simulink model "Indexer"  (R2018b)
settings: Solver=ode1  StartTime=0.0  StopTime=10.0  FixedStep=0.001  RelTol=1e-3
undefined symbols (not defined in the file): world
libraries: simulink x7
settings Model: Creator=ogihara  LastModifiedBy=ogihara

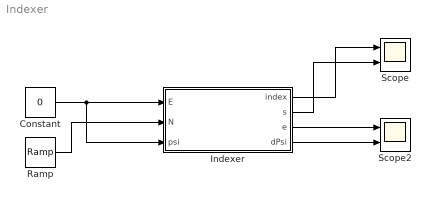
== system Indexer ==
  Constant : Constant  Value=0
  Indexer : Subsystem
  Ramp : simulink/Sources/Ramp  slope=10  start=0  InitialOutput=0
  Scope : Scope  NumInputPorts=2
  Scope2 : Scope  NumInputPorts=2
  wires:
  Constant/1 -> Indexer/3(psi), Indexer/1(E)
  Ramp/1 -> Indexer/2(N)
  Indexer/3(e) -> Scope2/1
  Indexer/4(dPsi) -> Scope2/2
  Indexer/1(index) -> Scope/1
  Indexer/2(s) -> Scope/2

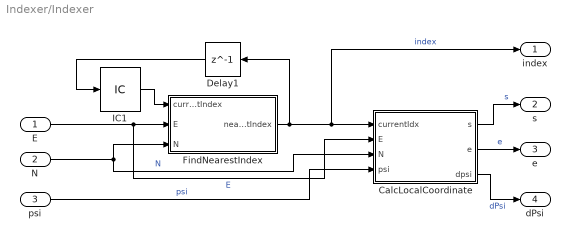
== system Indexer/Indexer ==
  E : Inport
  N : Inport  Port=2
  psi : Inport  Port=3
  CalcLocalCoordinate : Subsystem
  Delay1 : Delay  DelayLength=1
  FindNearestIndex : Subsystem
  IC1 : InitialCondition
  index : Outport
  s : Outport  Port=2
  e : Outport  Port=3
  dPsi : Outport  Port=4
  wires:
  IC1/1 -> FindNearestIndex/1(currentIndex)
  CalcLocalCoordinate/3(dpsi) -> dPsi/1  "dPsi"
  FindNearestIndex/1(nearestIndex) -> index/1, CalcLocalCoordinate/1(currentIdx), Delay1/1  "index"
  psi/1 -> CalcLocalCoordinate/4(psi)  "psi"
  E/1 -> CalcLocalCoordinate/2(E), FindNearestIndex/2(E)  "E"
  Delay1/1 -> IC1/1
  CalcLocalCoordinate/1(s) -> s/1  "s"
  N/1 -> CalcLocalCoordinate/3(N), FindNearestIndex/3(N)  "N"
  CalcLocalCoordinate/2(e) -> e/1  "e"

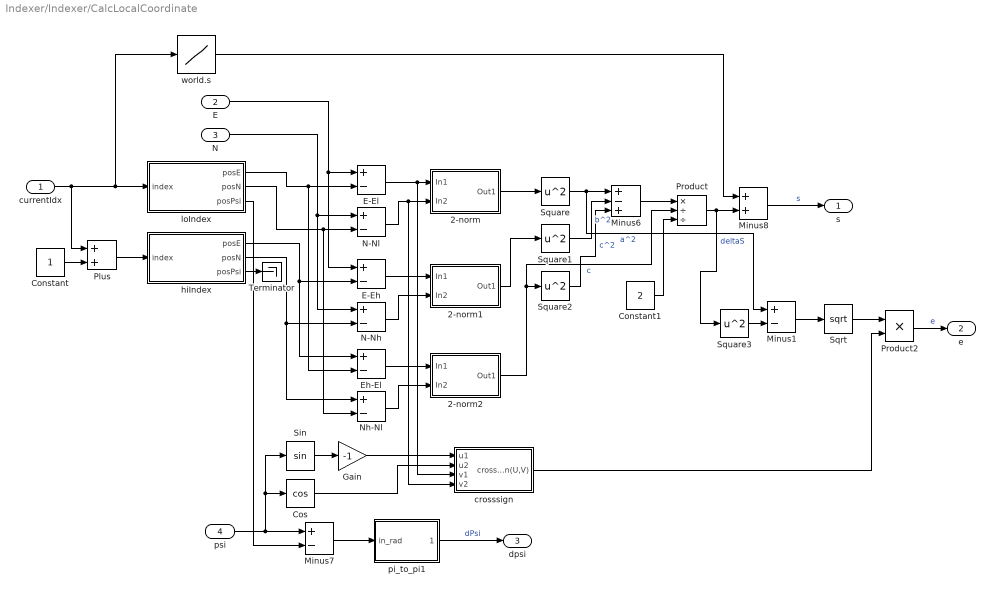
== system Indexer/Indexer/CalcLocalCoordinate ==
  currentIdx : Inport
  E : Inport  Port=2
  N : Inport  Port=3
  psi : Inport  Port=4
  2-norm : Subsystem
  2-norm1 : Subsystem
  2-norm2 : Subsystem
  Constant : Constant
  Constant1 : Constant  Value=2
  Cos : Trigonometry  Operator=cos
  E-Eh : Sum  Inputs=+-
  E-El : Sum  Inputs=+-
  Eh-El : Sum  Inputs=+-
  Gain : Gain  Gain=-1
  Minus1 : Sum  Inputs=+-
  Minus6 : Sum  Inputs=+-+
  Minus7 : Sum  Inputs=+-
  Minus8 : Sum
  N-Nh : Sum  Inputs=+-
  N-Nl : Sum  Inputs=+-
  Nh-Nl : Sum  Inputs=+-
  Plus : Sum
  Product : Product  Inputs=*//
  Product2 : Product
  Sin : Trigonometry
  Sqrt : Sqrt  SaturateOnIntegerOverflow=on
  Square{,1..3} (4 alike) : Math  Operator=square  SaturateOnIntegerOverflow=on
  Terminator : Terminator
  crosssign : Subsystem
  hiIndex : Subsystem
  loIndex : Subsystem
  pi_to_pi1 : Subsystem
  world.s : Lookup_n-D  NumberOfTableDimensions=1  BreakpointsForDimension1=world.index  Table=world.s_m  InternalRulePriority=Speed  RndMeth=Simplest  InputSameDT=on
  s : Outport
  e : Outport  Port=2
  dpsi : Outport  Port=3
  wires:
  currentIdx/1 -> Plus/1, world.s/1, loIndex/1(index)
  Constant/1 -> Plus/2
  Plus/1 -> hiIndex/1(index)
  hiIndex/3(posPsi) -> Terminator/1
  hiIndex/1(posE) -> Eh-El/1, E-Eh/2
  E-El/1 -> crosssign/3(v1), 2-norm/1(In1)
  N-Nl/1 -> crosssign/4(v2), 2-norm/2(In2)
  E-Eh/1 -> 2-norm1/1(In1)
  N-Nh/1 -> 2-norm1/2(In2)
  Eh-El/1 -> 2-norm2/1(In1)
  Nh-Nl/1 -> 2-norm2/2(In2)
  2-norm/1(Out1) -> Square/1
  2-norm1/1(Out1) -> Square1/1
  2-norm2/1(Out1) -> Product/2, Square2/1  "c"
  Square/1 -> Minus1/1, Minus6/1  "a^2"
  Square1/1 -> Minus6/2  "b^2"
  Square2/1 -> Minus6/3  "c^2"
  Minus6/1 -> Product/1
  Constant1/1 -> Product/3
  psi/1 -> Cos/1, Sin/1, Minus7/1
  Minus7/1 -> pi_to_pi1/1(in_rad)
  Product/1 -> Square3/1, Minus8/2  "deltaS"
  world.s/1 -> Minus8/1
  Minus8/1 -> s/1  "s"
  Sin/1 -> Gain/1
  Gain/1 -> crosssign/1(u1)
  Cos/1 -> crosssign/2(u2)
  E/1 -> E-Eh/1, E-El/1
  loIndex/1(posE) -> Eh-El/2, E-El/2
  loIndex/2(posN) -> Nh-Nl/2, N-Nl/2
  N/1 -> N-Nh/1, N-Nl/1
  hiIndex/2(posN) -> Nh-Nl/1, N-Nh/2
  loIndex/3(posPsi) -> Minus7/2
  Square3/1 -> Minus1/2
  Minus1/1 -> Sqrt/1
  Sqrt/1 -> Product2/1
  Product2/1 -> e/1  "e"
  crosssign/1(crosssign(U,V)) -> Product2/2
  pi_to_pi1/1(out_rad) -> dpsi/1  "dPsi"

== system Indexer/Indexer/FindNearestIndex ==
  note: Osprey had forward & backward search.
      | This simulator has only forward search and max width is 5.
  currentIndex : Inport
  E : Inport  Port=2
  N : Inport  Port=3
  ForwardSearch : Subsystem  TreatAsAtomicUnit=on
  nearestIndex : Outport
  wires:
  currentIndex/1 -> ForwardSearch/1(CurrentIndex)
  E/1 -> ForwardSearch/2(E)
  N/1 -> ForwardSearch/3(N)
  ForwardSearch/1(loIndexF) -> nearestIndex/1

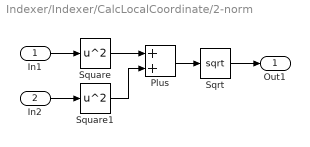
== system Indexer/Indexer/CalcLocalCoordinate/2-norm ==
  In1 : Inport
  In2 : Inport  Port=2
  Plus : Sum
  Sqrt : Sqrt  SaturateOnIntegerOverflow=on
  Square : Math  Operator=square  SaturateOnIntegerOverflow=on
  Square1 : Math  Operator=square  SaturateOnIntegerOverflow=on
  Out1 : Outport
  wires:
  In1/1 -> Square/1
  In2/1 -> Square1/1
  Square/1 -> Plus/1
  Square1/1 -> Plus/2
  Plus/1 -> Sqrt/1
  Sqrt/1 -> Out1/1

== system Indexer/Indexer/CalcLocalCoordinate/2-norm1 ==
  In1 : Inport
  In2 : Inport  Port=2
  Plus : Sum
  Sqrt : Sqrt  SaturateOnIntegerOverflow=on
  Square : Math  Operator=square  SaturateOnIntegerOverflow=on
  Square1 : Math  Operator=square  SaturateOnIntegerOverflow=on
  Out1 : Outport
  wires:
  In1/1 -> Square/1
  In2/1 -> Square1/1
  Square/1 -> Plus/1
  Square1/1 -> Plus/2
  Plus/1 -> Sqrt/1
  Sqrt/1 -> Out1/1

== system Indexer/Indexer/CalcLocalCoordinate/2-norm2 ==
  In1 : Inport
  In2 : Inport  Port=2
  Plus : Sum
  Sqrt : Sqrt  SaturateOnIntegerOverflow=on
  Square : Math  Operator=square  SaturateOnIntegerOverflow=on
  Square1 : Math  Operator=square  SaturateOnIntegerOverflow=on
  Out1 : Outport
  wires:
  In1/1 -> Square/1
  In2/1 -> Square1/1
  Square/1 -> Plus/1
  Square1/1 -> Plus/2
  Plus/1 -> Sqrt/1
  Sqrt/1 -> Out1/1

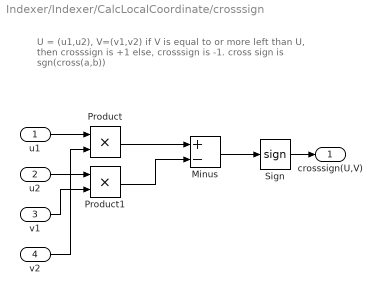
== system Indexer/Indexer/CalcLocalCoordinate/crosssign ==
  note: U = (u1,u2), V=(v1,v2)
      | if V is equal to or more left than U, then crosssign is +1
      | else, crosssign is -1.
      |
      | cross sign is sgn(cross(a,b))
  u1 : Inport
  u2 : Inport  Port=2
  v1 : Inport  Port=3
  v2 : Inport  Port=4
  Minus : Sum  Inputs=+-
  Product : Product
  Product1 : Product
  Sign : Signum
  crosssign(U,V) : Outport
  wires:
  Minus/1 -> Sign/1
  Sign/1 -> crosssign(U,V)/1
  u1/1 -> Product/1
  v2/1 -> Product/2
  u2/1 -> Product1/1
  v1/1 -> Product1/2
  Product/1 -> Minus/1
  Product1/1 -> Minus/2

== system Indexer/Indexer/CalcLocalCoordinate/hiIndex ==
  index : Inport
  world.posE_m : Lookup_n-D  NumberOfTableDimensions=1  BreakpointsForDimension1=world.index  Table=world.posE_m  InternalRulePriority=Speed  RndMeth=Simplest  InputSameDT=on
  world.posN_m : Lookup_n-D  NumberOfTableDimensions=1  BreakpointsForDimension1=world.index  Table=world.posN_m  InternalRulePriority=Speed  RndMeth=Simplest  InputSameDT=on
  world.psi_rad : Lookup_n-D  NumberOfTableDimensions=1  BreakpointsForDimension1=world.index  Table=world.psi_rad  InternalRulePriority=Speed  RndMeth=Simplest  InputSameDT=on
  posE : Outport
  posN : Outport  Port=2
  posPsi : Outport  Port=3
  wires:
  world.psi_rad/1 -> posPsi/1
  index/1 -> world.psi_rad/1, world.posN_m/1, world.posE_m/1
  world.posE_m/1 -> posE/1
  world.posN_m/1 -> posN/1

== system Indexer/Indexer/CalcLocalCoordinate/loIndex ==
  index : Inport
  world.posE_m : Lookup_n-D  NumberOfTableDimensions=1  BreakpointsForDimension1=world.index  Table=world.posE_m  InternalRulePriority=Speed  RndMeth=Simplest  InputSameDT=on
  world.posN_m : Lookup_n-D  NumberOfTableDimensions=1  BreakpointsForDimension1=world.index  Table=world.posN_m  InternalRulePriority=Speed  RndMeth=Simplest  InputSameDT=on
  world.psi_rad : Lookup_n-D  NumberOfTableDimensions=1  BreakpointsForDimension1=world.index  Table=world.psi_rad  InternalRulePriority=Speed  RndMeth=Simplest  InputSameDT=on
  posE : Outport
  posN : Outport  Port=2
  posPsi : Outport  Port=3
  wires:
  world.psi_rad/1 -> posPsi/1
  index/1 -> world.psi_rad/1, world.posN_m/1, world.posE_m/1
  world.posE_m/1 -> posE/1
  world.posN_m/1 -> posN/1

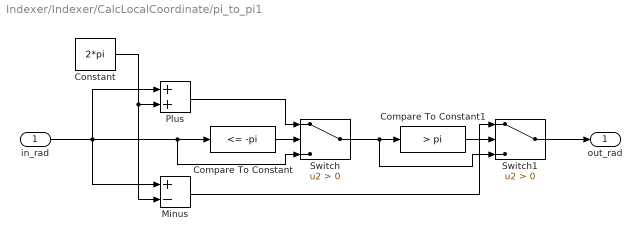
== system Indexer/Indexer/CalcLocalCoordinate/pi_to_pi1 ==
  in_rad : Inport
  Compare To Constant : simulink/Logic and Bit Operations/Compare To Constant  relop=<=  const=-pi  OutDataTypeStr=boolean
  Compare To Constant1 : simulink/Logic and Bit Operations/Compare To Constant  relop=>  const=pi  OutDataTypeStr=boolean
  Constant : Constant  Value=2*pi
  Minus : Sum  Inputs=+-
  Plus : Sum
  Switch : Switch  Criteria=u2 > Threshold
  Switch1 : Switch  Criteria=u2 > Threshold
  out_rad : Outport
  wires:
  Constant/1 -> Minus/2, Plus/2
  in_rad/1 -> Switch/3, Compare To Constant/1, Minus/1, Plus/1
  Compare To Constant1/1 -> Switch1/2
  Compare To Constant/1 -> Switch/2
  Plus/1 -> Switch/1
  Switch/1 -> Switch1/3, Compare To Constant1/1
  Minus/1 -> Switch1/1
  Switch1/1 -> out_rad/1

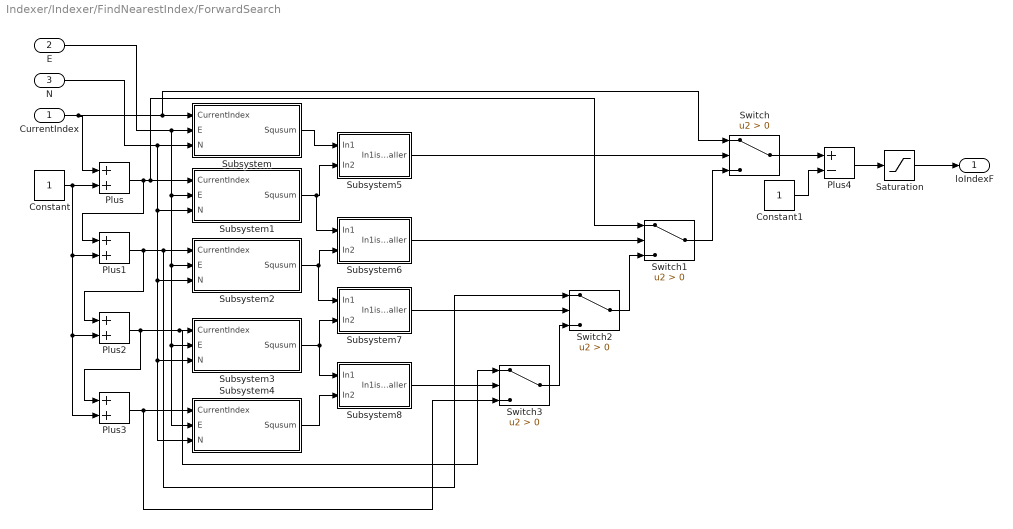
== system Indexer/Indexer/FindNearestIndex/ForwardSearch ==
  CurrentIndex : Inport
  E : Inport  Port=2
  N : Inport  Port=3
  Constant : Constant
  Constant1 : Constant
  Plus{,1..3} (4 alike) : Sum
  Plus4 : Sum  Inputs=+-
  Saturation : Saturate  UpperLimit=world.maxIndex  LowerLimit=1
  Subsystem : Subsystem
  Subsystem1 : Subsystem
  Subsystem2 : Subsystem
  Subsystem3 : Subsystem
  Subsystem4 : Subsystem
  Subsystem5 : Subsystem
  Subsystem6 : Subsystem
  Subsystem7 : Subsystem
  Subsystem8 : Subsystem
  Switch{,1..3} (4 alike) : Switch  Criteria=u2 > Threshold
  loIndexF : Outport
  wires:
  Constant/1 -> Plus2/2, Plus3/2, Plus1/2, Plus/2
  CurrentIndex/1 -> Plus/1, Switch/1, Subsystem/1(CurrentIndex)
  Plus/1 -> Subsystem1/1(CurrentIndex), Switch1/1, Plus1/1
  E/1 -> Subsystem1/2(E), Subsystem2/2(E), Subsystem4/2(E), Subsystem3/2(E), Subsystem/2(E)
  N/1 -> Subsystem1/3(N), Subsystem2/3(N), Subsystem4/3(N), Subsystem3/3(N), Subsystem/3(N)
  Plus1/1 -> Plus2/1, Subsystem2/1(CurrentIndex), Switch2/1
  Plus2/1 -> Switch3/1, Subsystem3/1(CurrentIndex), Plus3/1
  Subsystem/1(Squsum) -> Subsystem5/1(In1)
  Subsystem1/1(Squsum) -> Subsystem6/1(In1), Subsystem5/2(In2)
  Subsystem2/1(Squsum) -> Subsystem7/1(In1), Subsystem6/2(In2)
  Subsystem3/1(Squsum) -> Subsystem8/1(In1), Subsystem7/2(In2)
  Subsystem4/1(Squsum) -> Subsystem8/2(In2)
  Subsystem5/1(In1isSmaller) -> Switch/2
  Subsystem6/1(In1isSmaller) -> Switch1/2
  Subsystem7/1(In1isSmaller) -> Switch2/2
  Subsystem8/1(In1isSmaller) -> Switch3/2
  Switch/1 -> Plus4/1
  Switch1/1 -> Switch/3
  Switch2/1 -> Switch1/3
  Switch3/1 -> Switch2/3
  Plus3/1 -> Subsystem4/1(CurrentIndex), Switch3/3
  Plus4/1 -> Saturation/1
  Saturation/1 -> loIndexF/1
  Constant1/1 -> Plus4/2

== system Indexer/Indexer/FindNearestIndex/ForwardSearch/Subsystem ==
  CurrentIndex : Inport
  E : Inport  Port=2
  N : Inport  Port=3
  Saturation : Saturate  UpperLimit=world.maxIndex  LowerLimit=1
  squaresum : Subsystem
  world : Subsystem
  Squsum : Outport
  wires:
  squaresum/1(squsum) -> Squsum/1
  CurrentIndex/1 -> Saturation/1
  N/1 -> squaresum/4(N2)
  world/1(posE) -> squaresum/1(E1)
  E/1 -> squaresum/3(E2)
  world/2(posN) -> squaresum/2(N1)
  Saturation/1 -> world/1(index)

== system Indexer/Indexer/FindNearestIndex/ForwardSearch/Subsystem1 ==
  CurrentIndex : Inport
  E : Inport  Port=2
  N : Inport  Port=3
  Saturation : Saturate  UpperLimit=world.maxIndex  LowerLimit=1
  squaresum : Subsystem
  world : Subsystem
  Squsum : Outport
  wires:
  squaresum/1(squsum) -> Squsum/1
  CurrentIndex/1 -> Saturation/1
  N/1 -> squaresum/4(N2)
  world/1(posE) -> squaresum/1(E1)
  E/1 -> squaresum/3(E2)
  world/2(posN) -> squaresum/2(N1)
  Saturation/1 -> world/1(index)

== system Indexer/Indexer/FindNearestIndex/ForwardSearch/Subsystem2 ==
  CurrentIndex : Inport
  E : Inport  Port=2
  N : Inport  Port=3
  Saturation : Saturate  UpperLimit=world.maxIndex  LowerLimit=1
  squaresum : Subsystem
  world : Subsystem
  Squsum : Outport
  wires:
  squaresum/1(squsum) -> Squsum/1
  CurrentIndex/1 -> Saturation/1
  N/1 -> squaresum/4(N2)
  world/1(posE) -> squaresum/1(E1)
  E/1 -> squaresum/3(E2)
  world/2(posN) -> squaresum/2(N1)
  Saturation/1 -> world/1(index)

== system Indexer/Indexer/FindNearestIndex/ForwardSearch/Subsystem3 ==
  CurrentIndex : Inport
  E : Inport  Port=2
  N : Inport  Port=3
  Saturation : Saturate  UpperLimit=world.maxIndex  LowerLimit=1
  squaresum : Subsystem
  world : Subsystem
  Squsum : Outport
  wires:
  squaresum/1(squsum) -> Squsum/1
  CurrentIndex/1 -> Saturation/1
  N/1 -> squaresum/4(N2)
  world/1(posE) -> squaresum/1(E1)
  E/1 -> squaresum/3(E2)
  world/2(posN) -> squaresum/2(N1)
  Saturation/1 -> world/1(index)

== system Indexer/Indexer/FindNearestIndex/ForwardSearch/Subsystem4 ==
  CurrentIndex : Inport
  E : Inport  Port=2
  N : Inport  Port=3
  Saturation : Saturate  UpperLimit=world.maxIndex  LowerLimit=1
  squaresum : Subsystem
  world : Subsystem
  Squsum : Outport
  wires:
  squaresum/1(squsum) -> Squsum/1
  CurrentIndex/1 -> Saturation/1
  N/1 -> squaresum/4(N2)
  world/1(posE) -> squaresum/1(E1)
  E/1 -> squaresum/3(E2)
  world/2(posN) -> squaresum/2(N1)
  Saturation/1 -> world/1(index)

== system Indexer/Indexer/FindNearestIndex/ForwardSearch/Subsystem5 ==
  In1 : Inport
  In2 : Inport  Port=2
  Compare To Zero : simulink/Logic and Bit Operations/Compare To Zero  relop=<  OutDataTypeStr=boolean
  Minus : Sum  Inputs=+-
  In1isSmaller : Outport
  wires:
  In1/1 -> Minus/1
  In2/1 -> Minus/2
  Minus/1 -> Compare To Zero/1
  Compare To Zero/1 -> In1isSmaller/1

== system Indexer/Indexer/FindNearestIndex/ForwardSearch/Subsystem6 ==
  In1 : Inport
  In2 : Inport  Port=2
  Compare To Zero : simulink/Logic and Bit Operations/Compare To Zero  relop=<  OutDataTypeStr=boolean
  Minus : Sum  Inputs=+-
  In1isSmaller : Outport
  wires:
  In1/1 -> Minus/1
  In2/1 -> Minus/2
  Minus/1 -> Compare To Zero/1
  Compare To Zero/1 -> In1isSmaller/1

== system Indexer/Indexer/FindNearestIndex/ForwardSearch/Subsystem7 ==
  In1 : Inport
  In2 : Inport  Port=2
  Compare To Zero : simulink/Logic and Bit Operations/Compare To Zero  relop=<  OutDataTypeStr=boolean
  Minus : Sum  Inputs=+-
  In1isSmaller : Outport
  wires:
  In1/1 -> Minus/1
  In2/1 -> Minus/2
  Minus/1 -> Compare To Zero/1
  Compare To Zero/1 -> In1isSmaller/1

== system Indexer/Indexer/FindNearestIndex/ForwardSearch/Subsystem8 ==
  In1 : Inport
  In2 : Inport  Port=2
  Compare To Zero : simulink/Logic and Bit Operations/Compare To Zero  relop=<  OutDataTypeStr=boolean
  Minus : Sum  Inputs=+-
  In1isSmaller : Outport
  wires:
  In1/1 -> Minus/1
  In2/1 -> Minus/2
  Minus/1 -> Compare To Zero/1
  Compare To Zero/1 -> In1isSmaller/1

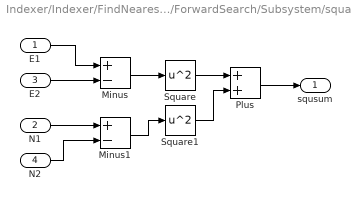
== system Indexer/Indexer/FindNearestIndex/ForwardSearch/Subsystem/squaresum ==
  E1 : Inport
  N1 : Inport  Port=2
  E2 : Inport  Port=3
  N2 : Inport  Port=4
  Minus : Sum  Inputs=+-
  Minus1 : Sum  Inputs=+-
  Plus : Sum
  Square : Math  Operator=square  SaturateOnIntegerOverflow=on
  Square1 : Math  Operator=square  SaturateOnIntegerOverflow=on
  squsum : Outport
  wires:
  N1/1 -> Minus1/1
  Minus/1 -> Square/1
  E1/1 -> Minus/1
  Plus/1 -> squsum/1
  Square1/1 -> Plus/2
  Minus1/1 -> Square1/1
  Square/1 -> Plus/1
  N2/1 -> Minus1/2
  E2/1 -> Minus/2

== system Indexer/Indexer/FindNearestIndex/ForwardSearch/Subsystem/world ==
  index : Inport
  world.posE_m : Lookup_n-D  NumberOfTableDimensions=1  BreakpointsForDimension1=world.index  Table=world.posE_m  InternalRulePriority=Speed  RndMeth=Simplest  InputSameDT=on
  world.posN_m : Lookup_n-D  NumberOfTableDimensions=1  BreakpointsForDimension1=world.index  Table=world.posN_m  InternalRulePriority=Speed  RndMeth=Simplest  InputSameDT=on
  posE : Outport
  posN : Outport  Port=2
  wires:
  index/1 -> world.posN_m/1, world.posE_m/1
  world.posE_m/1 -> posE/1
  world.posN_m/1 -> posN/1

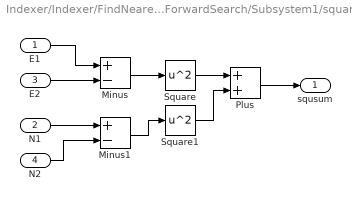
== system Indexer/Indexer/FindNearestIndex/ForwardSearch/Subsystem1/squaresum ==
  E1 : Inport
  N1 : Inport  Port=2
  E2 : Inport  Port=3
  N2 : Inport  Port=4
  Minus : Sum  Inputs=+-
  Minus1 : Sum  Inputs=+-
  Plus : Sum
  Square : Math  Operator=square  SaturateOnIntegerOverflow=on
  Square1 : Math  Operator=square  SaturateOnIntegerOverflow=on
  squsum : Outport
  wires:
  N1/1 -> Minus1/1
  Minus/1 -> Square/1
  E1/1 -> Minus/1
  Plus/1 -> squsum/1
  Square1/1 -> Plus/2
  Minus1/1 -> Square1/1
  Square/1 -> Plus/1
  N2/1 -> Minus1/2
  E2/1 -> Minus/2

== system Indexer/Indexer/FindNearestIndex/ForwardSearch/Subsystem1/world ==
  index : Inport
  world.posE_m : Lookup_n-D  NumberOfTableDimensions=1  BreakpointsForDimension1=world.index  Table=world.posE_m  InternalRulePriority=Speed  RndMeth=Simplest  InputSameDT=on
  world.posN_m : Lookup_n-D  NumberOfTableDimensions=1  BreakpointsForDimension1=world.index  Table=world.posN_m  InternalRulePriority=Speed  RndMeth=Simplest  InputSameDT=on
  posE : Outport
  posN : Outport  Port=2
  wires:
  index/1 -> world.posN_m/1, world.posE_m/1
  world.posE_m/1 -> posE/1
  world.posN_m/1 -> posN/1

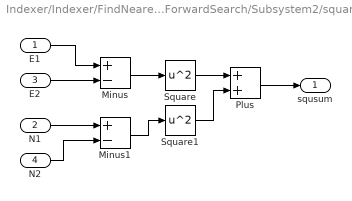
== system Indexer/Indexer/FindNearestIndex/ForwardSearch/Subsystem2/squaresum ==
  E1 : Inport
  N1 : Inport  Port=2
  E2 : Inport  Port=3
  N2 : Inport  Port=4
  Minus : Sum  Inputs=+-
  Minus1 : Sum  Inputs=+-
  Plus : Sum
  Square : Math  Operator=square  SaturateOnIntegerOverflow=on
  Square1 : Math  Operator=square  SaturateOnIntegerOverflow=on
  squsum : Outport
  wires:
  N1/1 -> Minus1/1
  Minus/1 -> Square/1
  E1/1 -> Minus/1
  Plus/1 -> squsum/1
  Square1/1 -> Plus/2
  Minus1/1 -> Square1/1
  Square/1 -> Plus/1
  N2/1 -> Minus1/2
  E2/1 -> Minus/2

== system Indexer/Indexer/FindNearestIndex/ForwardSearch/Subsystem2/world ==
  index : Inport
  world.posE_m : Lookup_n-D  NumberOfTableDimensions=1  BreakpointsForDimension1=world.index  Table=world.posE_m  InternalRulePriority=Speed  RndMeth=Simplest  InputSameDT=on
  world.posN_m : Lookup_n-D  NumberOfTableDimensions=1  BreakpointsForDimension1=world.index  Table=world.posN_m  InternalRulePriority=Speed  RndMeth=Simplest  InputSameDT=on
  posE : Outport
  posN : Outport  Port=2
  wires:
  index/1 -> world.posN_m/1, world.posE_m/1
  world.posE_m/1 -> posE/1
  world.posN_m/1 -> posN/1

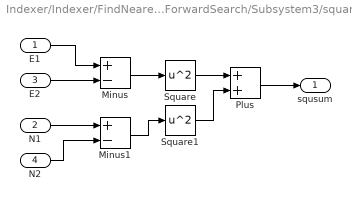
== system Indexer/Indexer/FindNearestIndex/ForwardSearch/Subsystem3/squaresum ==
  E1 : Inport
  N1 : Inport  Port=2
  E2 : Inport  Port=3
  N2 : Inport  Port=4
  Minus : Sum  Inputs=+-
  Minus1 : Sum  Inputs=+-
  Plus : Sum
  Square : Math  Operator=square  SaturateOnIntegerOverflow=on
  Square1 : Math  Operator=square  SaturateOnIntegerOverflow=on
  squsum : Outport
  wires:
  N1/1 -> Minus1/1
  Minus/1 -> Square/1
  E1/1 -> Minus/1
  Plus/1 -> squsum/1
  Square1/1 -> Plus/2
  Minus1/1 -> Square1/1
  Square/1 -> Plus/1
  N2/1 -> Minus1/2
  E2/1 -> Minus/2

== system Indexer/Indexer/FindNearestIndex/ForwardSearch/Subsystem3/world ==
  index : Inport
  world.posE_m : Lookup_n-D  NumberOfTableDimensions=1  BreakpointsForDimension1=world.index  Table=world.posE_m  InternalRulePriority=Speed  RndMeth=Simplest  InputSameDT=on
  world.posN_m : Lookup_n-D  NumberOfTableDimensions=1  BreakpointsForDimension1=world.index  Table=world.posN_m  InternalRulePriority=Speed  RndMeth=Simplest  InputSameDT=on
  posE : Outport
  posN : Outport  Port=2
  wires:
  index/1 -> world.posN_m/1, world.posE_m/1
  world.posE_m/1 -> posE/1
  world.posN_m/1 -> posN/1

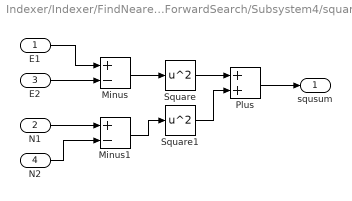
== system Indexer/Indexer/FindNearestIndex/ForwardSearch/Subsystem4/squaresum ==
  E1 : Inport
  N1 : Inport  Port=2
  E2 : Inport  Port=3
  N2 : Inport  Port=4
  Minus : Sum  Inputs=+-
  Minus1 : Sum  Inputs=+-
  Plus : Sum
  Square : Math  Operator=square  SaturateOnIntegerOverflow=on
  Square1 : Math  Operator=square  SaturateOnIntegerOverflow=on
  squsum : Outport
  wires:
  N1/1 -> Minus1/1
  Minus/1 -> Square/1
  E1/1 -> Minus/1
  Plus/1 -> squsum/1
  Square1/1 -> Plus/2
  Minus1/1 -> Square1/1
  Square/1 -> Plus/1
  N2/1 -> Minus1/2
  E2/1 -> Minus/2

== system Indexer/Indexer/FindNearestIndex/ForwardSearch/Subsystem4/world ==
  index : Inport
  world.posE_m : Lookup_n-D  NumberOfTableDimensions=1  BreakpointsForDimension1=world.index  Table=world.posE_m  InternalRulePriority=Speed  RndMeth=Simplest  InputSameDT=on
  world.posN_m : Lookup_n-D  NumberOfTableDimensions=1  BreakpointsForDimension1=world.index  Table=world.posN_m  InternalRulePriority=Speed  RndMeth=Simplest  InputSameDT=on
  posE : Outport
  posN : Outport  Port=2
  wires:
  index/1 -> world.posN_m/1, world.posE_m/1
  world.posE_m/1 -> posE/1
  world.posN_m/1 -> posN/1
